simulink model "Boeing787_NewMission_ElectricalThermal_2013"  (R2013a)
settings: Solver=ode23tb  SolverMode=SingleTasking  StartTime=0.0  StopTime=18000  RelTol=1e-3
InitFcn:
  | load('SampleOutput.mat')
  | 
  | load('SampleFuelBurn.mat')
StartFcn:
  | tic
StopFcn:
  | ttt = toc
  | tend = eval(get_param(bdroot,'StopTime'));
  | disp(['Total Simulation Time (s) = ' num2str(ttt) 's']);
  | RTR =  ttt/tend
  | disp(['Simulation Speed is ' num2str(tend/ttt) 'x faster than real-time']);
values from neighbouring files (symbols this model uses):
  CurrentMission = Mission(i)    [mission_plan.m]
  seed = 1    [mission_plan.m]
undefined symbols (not defined in the file or in its folder): FuelBurn
libraries: PowerFlowLib x17, simulink x12, powerlib_meascontrol x1
(part 1 of 17)
settings Model: Creator=Bradford  LastModifiedBy=caoyue
settings DataIOCC: SignalLoggingSaveFormat=ModelDataLogs
settings OptimizationCC: BlockReduction=off  BooleanDataType=off
settings DebuggingCC: SaveWithParameterizedLinksMsg=none  SignalResolutionControl=TryResolveAllWithWarning  SolverPrmCheckMsg=none  MultiTaskDSMMsg=warning  MultiTaskCondExecSysMsg=none  FrameProcessingCompatibilityMsg=error
settings HardwareCC: TargetUnknown=on
settings GRTTargetCC: CodeReplacementLibrary=C89/C90 (ANSI)

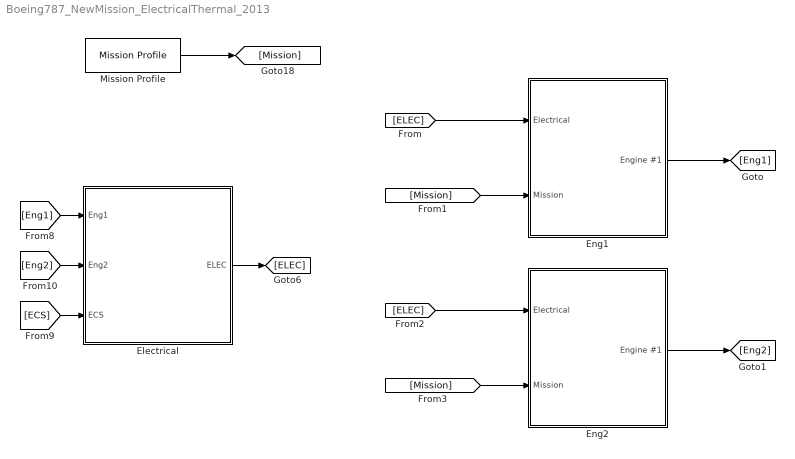
== system Boeing787_NewMission_ElectricalThermal_2013 ==
  Electrical : Subsystem
  Eng1 : Subsystem
  Eng2 : Subsystem
  Mission Profile : PowerFlowLib/Mission Profile/Mission Profile  mssn_check=off  mssn_prof=MSSN  del_P=0  del_T=0  del_rho=0  pres_msl=101.3  temp_msl=15  dens_msl=1.229
  wires:
  [ELEC] -> Eng1/1(Electrical)
  [Mission] -> Eng1/2(Mission)
  Eng1/1(Engine #1) -> [Eng1]
  Mission Profile/1 -> [Mission]
  [ELEC] -> Eng2/1(Electrical)
  [Mission] -> Eng2/2(Mission)
  Eng2/1(Engine #1) -> [Eng2]
  [Eng1] -> Electrical/1(Eng1)
  [ECS] -> Electrical/3(ECS)
  [Eng2] -> Electrical/2(Eng2)
  Electrical/1(ELEC) -> [ELEC]
